simulink model "mdl_bicycleModel_Integrator"  (R2019b)
settings: Solver=ode3  StartTime=0.0  StopTime=TotalTime  FixedStep=deltaT  MaxStep=deltaT  RelTol=1e-3  EnableMultiTasking=on
values from neighbouring files (symbols this model uses):
  a = vehicle(vehicle_i).a    [script_bicycleModel_Integrator.m]
  b = vehicle(vehicle_i).b    [script_bicycleModel_Integrator.m]
  Caf = vehicle(vehicle_i).Caf    [script_bicycleModel_Integrator.m]
  Car = vehicle(vehicle_i).Car    [script_bicycleModel_Integrator.m]
  Iz = vehicle(vehicle_i).Iz    [script_bicycleModel_Integrator.m]
  m = vehicle(vehicle_i).m    [script_bicycleModel_Integrator.m]
  Period = 3    [script_bicycleModel_Integrator.m]    (also in script_testBicycleModel.m; script_testBicycleModelWithODE.m)
  steering_amplitude_degrees = 2    [script_bicycleModel_Integrator.m]    (also in script_testBicycleModel.m; script_testBicycleModelWithODE.m)
  U = 20    [script_bicycleModel_Integrator.m]    (also in script_testBicycleModel.m; script_testBicycleModelWithODE.m)
settings Model: Creator=snb10  LastModifiedBy=prasa
settings DataIOCC: LimitDataPoints=on  SaveFormat=Array  SignalLoggingSaveFormat=ModelDataLogs  ReturnWorkspaceOutputs=off  SignalLoggingName=sigsOut
settings OptimizationCC: InitFltsAndDblsToZero=on  LifeSpan=inf
settings DebuggingCC: SaveWithParameterizedLinksMsg=none  UnderspecifiedInitializationDetection=Classic  MergeDetectMultiDrivingBlocksExec=none  SignalResolutionControl=TryResolveAllWithWarning  MultiTaskDSMMsg=warning  MultiTaskCondExecSysMsg=none  FcnCallInpInsideContextMsg=warning  StateNameClashWarn=warning  SFUnexpectedBacktrackingDiag=warning  SFNoUnconditionalDefaultTransitionDiag=warning  SFExecutionAtInitializationDiag=none  ArithmeticOperatorsInVariantConditions=warning
settings HardwareCC: ProdBitPerPointer=32  ProdBitPerSizeT=32  ProdBitPerPtrDiffT=32  ProdLargestAtomicFloat=None  ProdIntDivRoundTo=Undefined  ProdEndianess=Unspecified  ProdWordSize=32  ProdHWDeviceType=32-bit Generic  TargetUnknown=on
settings ModelReferenceCC: PropagateSignalLabelsOutOfModel=off
settings SFSimCC: SimUseLocalCustomCode=off  CustomCodeUndefinedFunction=UseInterfaceOnly
settings RTWCC: RTWUseLocalCustomCode=off
settings CodeAppCC: StateflowObjectComments=on
settings GRTTargetCC: TargetFcnLib=ansi_tfl_tmw.mat  TargetLangStandard=C89/C90 (ANSI)  CombineOutputUpdateFcns=off  GRTInterface=on
settings ConfigComp: CovMetricSettings=dw  CovSaveCumulativeToWorkspaceVar=on  CovSaveSingleToWorkspaceVar=on  CovExternalEMLEnable=off

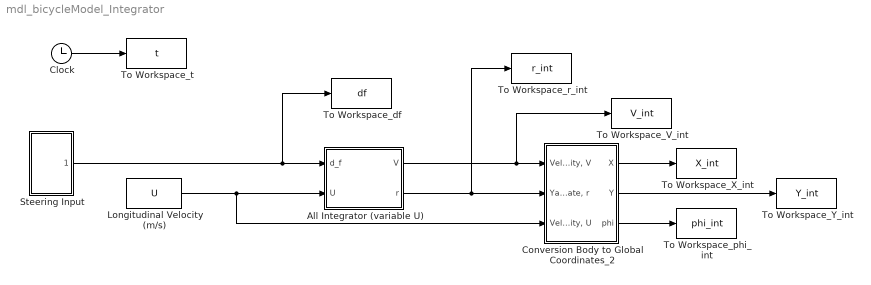
== system mdl_bicycleModel_Integrator ==
  All Integrator (variable U) : Subsystem
  Clock : Clock
  Conversion Body to Global Coordinates_2 : Subsystem
  Longitudinal Velocity (m/s) : Constant  Value=U
  Steering Input : Subsystem
  To Workspace_V_int : ToWorkspace  VariableName=V_int  SampleTime=-1
  To Workspace_X_int : ToWorkspace  VariableName=X_int  SampleTime=-1
  To Workspace_Y_int : ToWorkspace  VariableName=Y_int  SampleTime=-1
  To Workspace_df : ToWorkspace  VariableName=df  SampleTime=-1
  To Workspace_phi_int : ToWorkspace  VariableName=phi_int  SampleTime=-1
  To Workspace_r_int : ToWorkspace  VariableName=r_int  SampleTime=-1
  To Workspace_t : ToWorkspace  VariableName=t  SampleTime=-1
  wires:
  Clock/1 -> To Workspace_t/1
  All Integrator (variable U)/1(V) -> Conversion Body to Global Coordinates_2/1("Velocity, V"), To Workspace_V_int/1
  Conversion Body to Global Coordinates_2/1(X) -> To Workspace_X_int/1
  Conversion Body to Global Coordinates_2/2(Y) -> To Workspace_Y_int/1
  All Integrator (variable U)/2(r) -> Conversion Body to Global Coordinates_2/2("Yaw Rate, r"), To Workspace_r_int/1
  Conversion Body to Global Coordinates_2/3(phi) -> To Workspace_phi_int/1
  Longitudinal Velocity (m/s)/1 -> Conversion Body to Global Coordinates_2/3("Velocity, U"), All Integrator (variable U)/2(U)
  Steering Input/1(delta_f (radians)) -> To Workspace_df/1, All Integrator (variable U)/1(d_f)

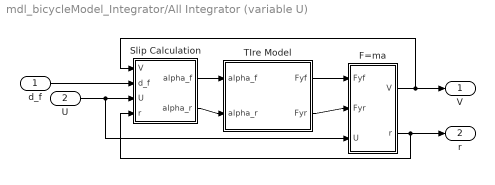
== system mdl_bicycleModel_Integrator/All Integrator (variable U) ==
  d_f : Inport
  U : Inport  Port=2
  F=ma : Subsystem
  Slip Calculation : Subsystem
  TIre Model : Subsystem
  V : Outport
  r : Outport  Port=2
  wires:
  Slip Calculation/1(alpha_f) -> TIre Model/1(alpha_f)
  Slip Calculation/2(alpha_r) -> TIre Model/2(alpha_r)
  TIre Model/1(Fyf) -> F=ma/1(Fyf)
  TIre Model/2(Fyr) -> F=ma/2(Fyr)
  U/1 -> Slip Calculation/3(U), F=ma/3(" U")
  d_f/1 -> Slip Calculation/2(d_f)
  F=ma/1(V) -> V/1, Slip Calculation/1(V)
  F=ma/2(r) -> r/1, Slip Calculation/4(r)

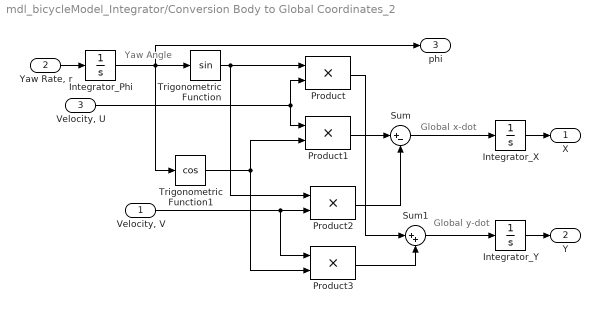
== system mdl_bicycleModel_Integrator/Conversion Body to Global Coordinates_2 ==
  note: Global y-dot
  note: Global x-dot
  note: Yaw Angle
  "Velocity, V" : Inport
  "Yaw Rate, r" : Inport  Port=2
  "Velocity, U" : Inport  Port=3
  Integrator_Phi : Integrator
  Integrator_X : Integrator
  Integrator_Y : Integrator
  Product{,1..3} (4 alike) : Product  SaturateOnIntegerOverflow=on  OutDataTypeStr=Inherit: Same as first input
  Sum : Sum  Inputs=|+-  SaturateOnIntegerOverflow=on
  Sum1 : Sum  Inputs=|++  SaturateOnIntegerOverflow=on
  Trigonometric Function : Trigonometry
  Trigonometric Function1 : Trigonometry  Operator=cos
  X : Outport
  Y : Outport  Port=2
  phi : Outport  Port=3
  wires:
  Integrator_Y/1 -> Y/1
  Integrator_X/1 -> X/1
  "Yaw Rate, r"/1 -> Integrator_Phi/1
  Sum1/1 -> Integrator_Y/1
  Product3/1 -> Sum1/2
  Product/1 -> Sum1/1
  Sum/1 -> Integrator_X/1
  Trigonometric Function/1 -> Product2/1, Product/1
  Product2/1 -> Sum/2
  Product1/1 -> Sum/1
  Trigonometric Function1/1 -> Product3/2, Product1/2
  "Velocity, V"/1 -> Product3/1, Product2/2
  "Velocity, U"/1 -> Product1/1, Product/2
  Integrator_Phi/1 -> phi/1, Trigonometric Function1/1, Trigonometric Function/1

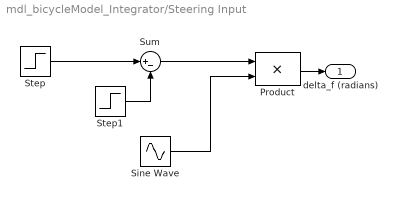
== system mdl_bicycleModel_Integrator/Steering Input ==
  Product : Product  SaturateOnIntegerOverflow=on  OutDataTypeStr=Inherit: Same as first input
  Sine Wave : Sin  Amplitude=steering_amplitude_degrees*pi/180  Frequency=2*pi/Period  SampleTime=0
  Step : Step  Time=0  SampleTime=0
  Step1 : Step  Time=Period  SampleTime=0
  Sum : Sum  Inputs=|+-  SaturateOnIntegerOverflow=on
  delta_f (radians) : Outport
  wires:
  Step/1 -> Sum/1
  Step1/1 -> Sum/2
  Sum/1 -> Product/1
  Sine Wave/1 -> Product/2
  Product/1 -> delta_f (radians)/1

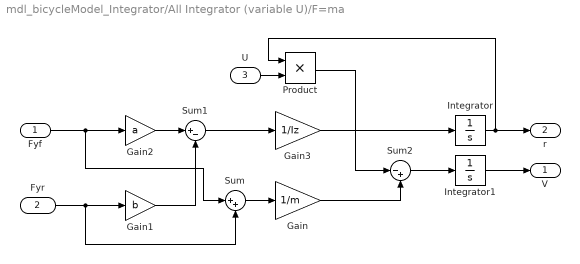
== system mdl_bicycleModel_Integrator/All Integrator (variable U)/F=ma ==
  Fyf : Inport
  Fyr : Inport  Port=2
  " U" : Inport  Port=3
  Gain : Gain  Gain=1/m
  Gain1 : Gain  Gain=b
  Gain2 : Gain  Gain=a
  Gain3 : Gain  Gain=1/Iz
  Integrator : Integrator
  Integrator1 : Integrator
  Product : Product  RndMeth=Zero
  Sum : Sum  Inputs=|++
  Sum1 : Sum  Inputs=|+-
  Sum2 : Sum  Inputs=|-+
  V : Outport
  r : Outport  Port=2
  wires:
  Fyf/1 -> Sum/1, Gain2/1
  Fyr/1 -> Sum/2, Gain1/1
  Gain2/1 -> Sum1/1
  Gain1/1 -> Sum1/2
  Sum1/1 -> Gain3/1
  Gain3/1 -> Integrator/1
  Sum/1 -> Gain/1
  Product/1 -> Sum2/1
  Gain/1 -> Sum2/2
  Sum2/1 -> Integrator1/1
  Integrator/1 -> r/1, Product/1
  Integrator1/1 -> V/1
  " U"/1 -> Product/2

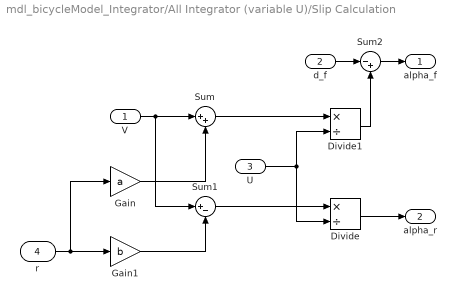
== system mdl_bicycleModel_Integrator/All Integrator (variable U)/Slip Calculation ==
  V : Inport
  d_f : Inport  Port=2
  U : Inport  Port=3
  r : Inport  Port=4
  Divide : Product  Inputs=*/
  Divide1 : Product  Inputs=*/
  Gain : Gain  Gain=a
  Gain1 : Gain  Gain=b
  Sum : Sum  Inputs=|++
  Sum1 : Sum  Inputs=|+-
  Sum2 : Sum  Inputs=|-+
  alpha_f : Outport
  alpha_r : Outport  Port=2
  wires:
  V/1 -> Sum/1, Sum1/1
  Gain/1 -> Sum/2
  r/1 -> Gain/1, Gain1/1
  Gain1/1 -> Sum1/2
  Sum/1 -> Divide1/1
  U/1 -> Divide1/2, Divide/2
  Sum1/1 -> Divide/1
  Divide1/1 -> Sum2/2
  d_f/1 -> Sum2/1
  Sum2/1 -> alpha_f/1
  Divide/1 -> alpha_r/1

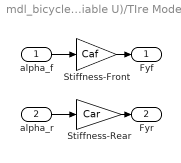
== system mdl_bicycleModel_Integrator/All Integrator (variable U)/TIre Model ==
  alpha_f : Inport
  alpha_r : Inport  Port=2
  Stiffness-Front : Gain  Gain=Caf
  Stiffness-Rear : Gain  Gain=Car
  Fyf : Outport
  Fyr : Outport  Port=2
  wires:
  alpha_f/1 -> Stiffness-Front/1
  Stiffness-Front/1 -> Fyf/1
  alpha_r/1 -> Stiffness-Rear/1
  Stiffness-Rear/1 -> Fyr/1
